simulink model "TKV"  (R2021a)
settings: Solver=VariableStepAuto  StartTime=0.0  StopTime=10.0  RelTol=1e-3
libraries: fuzblock x1
settings Model: Creator=Nobody  LastModifiedBy=Nobody

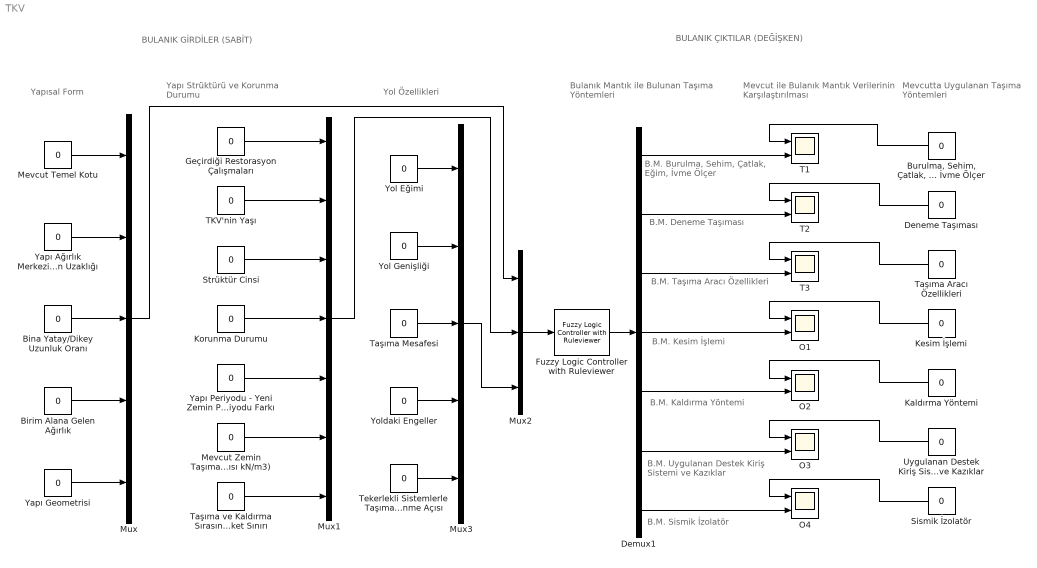
== system TKV ==
  note: Yapısal Form
  note: Yapı Strüktürü
      | ve Korunma Durumu
  note: Yol Özellikleri
  note: Bulanık Mantık ile Bulunan
      | Taşıma Yöntemleri
  note: Mevcutta Uygulanan
      | Taşıma Yöntemleri
  note: Mevcut ile Bulanık Mantık
      | Verilerinin Karşılaştırılması
  note: BULANIK GİRDİLER (SABİT)
  note: BULANIK ÇIKTILAR (DEĞİŞKEN)
  note: B.M. Burulma, Sehim,
      | Çatlak, Eğim, İvme Ölçer
  note: B.M. Deneme Taşıması
  note: B.M. Taşıma Aracı
      | Özellikleri
  note: B.M. Kesim İşlemi
  note: B.M. Kaldırma Yöntemi
  note: B.M. Uygulanan Destek
      | Kiriş Sistemi ve Kazıklar
  note: B.M. Sismik İzolatör
  Bina Yatay/Dikey Uzunluk Oranı : Constant  Value=0
  Birim Alana Gelen Ağırlık : Constant  Value=0
  "Burulma, Sehim, Çatlak, Eğim, İvme Ölçer" : Constant  Value=0
  Demux1 : Demux  Outputs=7
  Deneme Taşıması : Constant  Value=0
  Fuzzy Logic Controller with Ruleviewer : fuzblock/Fuzzy Logic  Controller  with Ruleviewer  fismatrix=fis  Ts=2
  Geçirdiği Restorasyon Çalışmaları : Constant  Value=0
  Kaldırma Yöntemi : Constant  Value=0
  Kesim İşlemi : Constant  Value=0
  Korunma Durumu : Constant  Value=0
  Mevcut Temel Kotu : Constant  Value=0
  Mevcut Zemin Taşıma Gücü (Yatak Katsayısı kN/m3) : Constant  Value=0
  Mux : Mux  Inputs=5
  Mux1 : Mux  Inputs=7
  Mux2 : Mux  Inputs=3
  Mux3 : Mux  Inputs=5
  O{1..4} (4 alike) : Scope  NumInputPorts=2
  Sismik İzolatör : Constant  Value=0
  Strüktür Cinsi : Constant  Value=0
  T1 : Scope  NumInputPorts=2
  T2 : Scope  NumInputPorts=2
  T3 : Scope  NumInputPorts=2
  TKV'nin Yaşı : Constant  Value=0
  Taşıma Aracı Özellikleri : Constant  Value=0
  Taşıma Mesafesi : Constant  Value=0
  Taşıma ve Kaldırma Sırasında Çatlaklarda İzin Verilen Hareket Sınırı : Constant  Value=0
  Tekerlekli Sistemlerle Taşımada Dönme Açısı : Constant  Value=0
  Uygulanan Destek Kiriş Sistemi ve Kazıklar : Constant  Value=0
  Yapı Ağırlık Merkezinin Rijitlik Merkezine Olan Uzaklığı : Constant  Value=0
  Yapı Geometrisi : Constant  Value=0
  Yapı Periyodu - Yeni Zemin Periyodu Farkı : Constant  Value=0
  Yol Eğimi : Constant  Value=0
  Yol Genişliği : Constant  Value=0
  Yoldaki Engeller : Constant  Value=0
  wires:
  Mevcut Temel Kotu/1 -> Mux/1
  Yapı Geometrisi/1 -> Mux/5
  Yapı Ağırlık Merkezinin Rijitlik Merkezine Olan Uzaklığı/1 -> Mux/2
  Bina Yatay/Dikey Uzunluk Oranı/1 -> Mux/3
  Birim Alana Gelen Ağırlık/1 -> Mux/4
  Korunma Durumu/1 -> Mux1/4
  Strüktür Cinsi/1 -> Mux1/3
  TKV'nin Yaşı/1 -> Mux1/2
  Yapı Periyodu - Yeni Zemin Periyodu Farkı/1 -> Mux1/5
  Geçirdiği Restorasyon Çalışmaları/1 -> Mux1/1
  Mux/1 -> Mux2/1
  Mux1/1 -> Mux2/2
  Mevcut Zemin Taşıma Gücü (Yatak Katsayısı kN/m3)/1 -> Mux1/6
  Taşıma ve Kaldırma Sırasında Çatlaklarda İzin Verilen Hareket Sınırı/1 -> Mux1/7
  Mux3/1 -> Mux2/3
  Yoldaki Engeller/1 -> Mux3/4
  Taşıma Mesafesi/1 -> Mux3/3
  Yol Genişliği/1 -> Mux3/2
  Tekerlekli Sistemlerle Taşımada Dönme Açısı/1 -> Mux3/5
  Yol Eğimi/1 -> Mux3/1
  Mux2/1 -> Fuzzy Logic Controller with Ruleviewer/1
  "Burulma, Sehim, Çatlak, Eğim, İvme Ölçer"/1 -> T1/1
  Demux1/1 -> T1/2
  Deneme Taşıması/1 -> T2/1
  Taşıma Aracı Özellikleri/1 -> T3/1
  Kesim İşlemi/1 -> O1/1
  Kaldırma Yöntemi/1 -> O2/1
  Uygulanan Destek Kiriş Sistemi ve Kazıklar/1 -> O3/1
  Sismik İzolatör/1 -> O4/1
  Demux1/2 -> T2/2
  Demux1/3 -> T3/2
  Demux1/4 -> O1/2
  Demux1/5 -> O2/2
  Demux1/6 -> O3/2
  Demux1/7 -> O4/2
  Fuzzy Logic Controller with Ruleviewer/1 -> Demux1/1
